simulink model "mEnabledModelVarSize"  (Simulink 8.0)
settings: Solver=FixedStepDiscrete  StartTime=0.0  StopTime=10.0  FixedStep=1  RelTol=1e-3
undefined symbols (not defined in the file or in its folder): j
settings Model: FPTRunName=Active  Creator=mtocci  LastModifiedBy=mtocci
settings DataIOCC: SignalLoggingSaveFormat=ModelDataLogs
settings OptimizationCC: InlineParams=on
settings DebuggingCC: FcnCallInpInsideContextMsg=Use local settings
settings ModelReferenceCC: ModelReferenceNumInstancesAllowed=Single  PropagateVarSize=During execution
settings GRTTargetCC: CombineOutputUpdateFcns=off

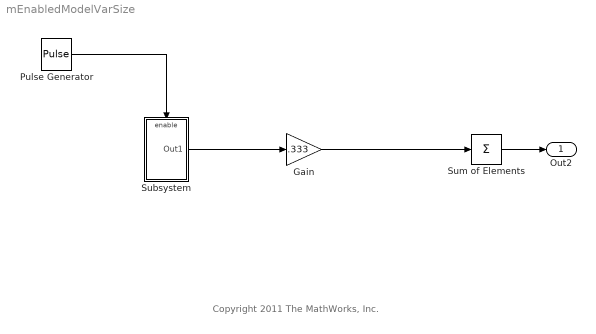
== system mEnabledModelVarSize ==
  note: Copyright 2011 The MathWorks, Inc.
  Gain : Gain  Gain=.333
  Pulse Generator : DiscretePulseGenerator
  Subsystem : Subsystem
  Sum of Elements : Sum  Inputs=+
  Out2 : Outport  InitialOutput=0
  wires:
  Gain/1 -> Sum of Elements/1
  Pulse Generator/1 -> Subsystem/Enable
  Subsystem/1(Out1) -> Gain/1
  Sum of Elements/1 -> Out2/1

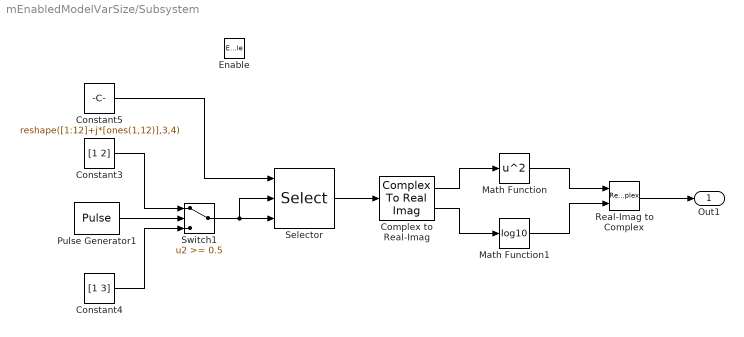
== system mEnabledModelVarSize/Subsystem ==
  Enable : EnablePort  PropagateVarSize=During execution  SampleTime=1
  Complex to Real-Imag : ComplexToRealImag
  Constant3 : Constant  Value=[1 2]
  Constant4 : Constant  Value=[1 3]
  Constant5 : Constant  Value=reshape([1:12]+j*[ones(1,12)],3,4)
  Math Function : Math  Operator=square  SaturateOnIntegerOverflow=on
  Math Function1 : Math  Operator=log10  SaturateOnIntegerOverflow=on
  Pulse Generator1 : DiscretePulseGenerator  Period=4  PulseWidth=2
  Real-Imag to Complex : RealImagToComplex
  Selector : Selector  NumberOfDimensions=2  InputPortWidth=3  IndexOptions=Starting and ending indices (port),Starting and ending indices (port)  Indices=[1 3],1  OutputSizes=1,1
  Switch1 : Switch  Threshold=0.5
  Out1 : Outport
  wires:
  Complex to Real-Imag/1 -> Math Function/1
  Math Function/1 -> Real-Imag to Complex/1
  Complex to Real-Imag/2 -> Math Function1/1
  Math Function1/1 -> Real-Imag to Complex/2
  Real-Imag to Complex/1 -> Out1/1
  Selector/1 -> Complex to Real-Imag/1
  Constant5/1 -> Selector/1
  Switch1/1 -> Selector/2, Selector/3
  Constant4/1 -> Switch1/3
  Pulse Generator1/1 -> Switch1/2
  Constant3/1 -> Switch1/1
